simulink model "opalWebSrvExp"  (Simulink 7.8)
settings: Solver=ode4  SolverMode=SingleTasking  StartTime=0  StopTime=inf  FixedStep=Tsrt  MaxStep=0.01  RelTol=1e-3  AbsTol=1e-6
PreLoadFcn:
  | Tsrt=5e-5;
  | Tscom=1e-2;
undefined symbols (not defined in the file): another_event_name, IP, my_event_name, UDP
libraries: rtlab x7, rtio_opalrt_op5142ex1 x5, rtio_generic_ip x1, powerlib_extras x1
settings Model: Creator=jwu  LastModifiedBy=Administrateur  ExtModeTrigMode=oneshot  ExtModeArmWhenConnect=off  BufferReuse=off
settings DataIOCC: ExternalInput=[]  InitialState=[]  LimitDataPoints=off  SaveOutput=off  SaveTime=off  SignalLoggingName=sigsOut
settings OptimizationCC: BooleanDataType=off  OptimizeBlockIOStorage=off  BufferReuse=off  ExpressionFolding=off  FoldNonRolledExpr=off  LocalBlockOutputs=off  InitFltsAndDblsToZero=on
settings DebuggingCC: SaveWithParameterizedLinksMsg=none  SignalResolutionControl=TryResolveAllWithWarning  SolverPrmCheckMsg=none  InheritedTsInSrcMsg=none  MultiTaskDSMMsg=warning  MultiTaskCondExecSysMsg=none  FcnCallInpInsideContextMsg=Use local settings  StrictBusMsg=None
settings HardwareCC: TargetUnknown=on
settings RTWCC: IncludeERTFirstTime=on
settings CodeAppCC: IgnoreCustomStorageClasses=off
settings GRTTargetCC: TargetFcnLib=ansi_tfl_tmw.mat

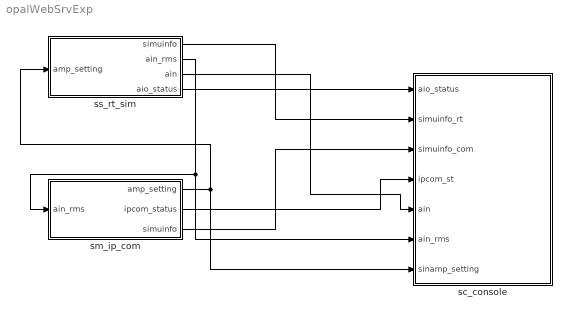
== system opalWebSrvExp ==
  sc_console : Subsystem
  sm_ip_com : Subsystem
  ss_rt_sim : Subsystem
  wires:
  ss_rt_sim/1(simuinfo) -> sc_console/2(simuinfo_rt)
  sm_ip_com/3(simuinfo) -> sc_console/3(simuinfo_com)
  ss_rt_sim/2(ain_rms) -> sm_ip_com/1(ain_rms), sc_console/6(ain_rms)
  sm_ip_com/1(amp_setting) -> ss_rt_sim/1(amp_setting), sc_console/7(sinamp_setting)
  ss_rt_sim/4(aio_status) -> sc_console/1(aio_status)
  sm_ip_com/2(ipcom_status) -> sc_console/4(ipcom_st)
  ss_rt_sim/3(ain) -> sc_console/5(ain)

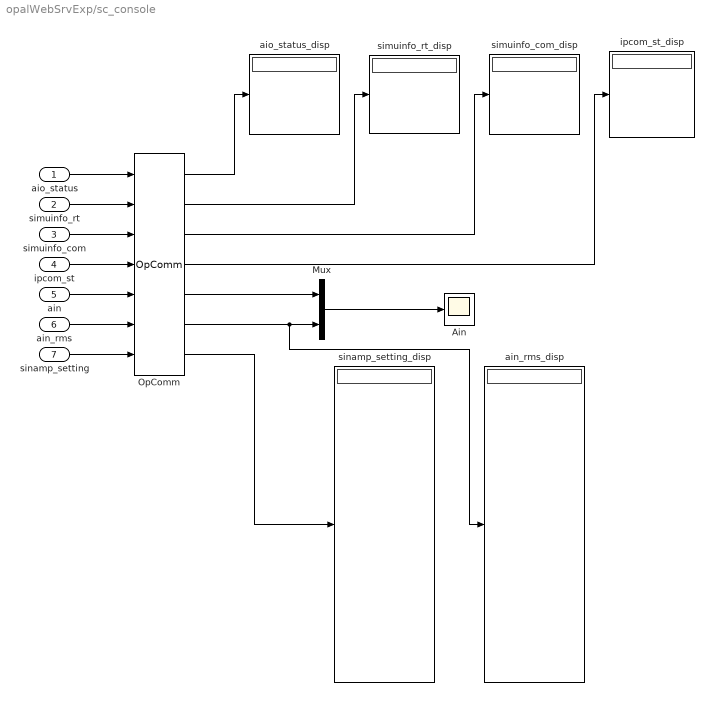
== system opalWebSrvExp/sc_console ==
  aio_status : Inport
  simuinfo_rt : Inport  Port=2
  simuinfo_com : Inport  Port=3
  ipcom_st : Inport  Port=4
  ain : Inport  Port=5
  ain_rms : Inport  Port=6
  sinamp_setting : Inport  Port=7
  Ain : Scope
  Mux : Mux  Inputs=2
  OpComm : rtlab/OpComm  nbport=7  groupe_acq=1  subsys_rate=0  st=0  Synchronization=on  Interpolation=on  Threshold=1.0  Missed_Data=off  Sim_Time=off  Samples=off  dynSigOut=off  from_console=0  warning_done=off  writeOpCommFile=off  Offset=off
  ain_rms_disp : Display
  aio_status_disp : Display
  ipcom_st_disp : Display
  simuinfo_com_disp : Display
  simuinfo_rt_disp : Display
  sinamp_setting_disp : Display
  wires:
  aio_status/1 -> OpComm/1
  ain/1 -> OpComm/5
  OpComm/1 -> aio_status_disp/1
  simuinfo_rt/1 -> OpComm/2
  simuinfo_com/1 -> OpComm/3
  OpComm/2 -> simuinfo_rt_disp/1
  OpComm/3 -> simuinfo_com_disp/1
  ipcom_st/1 -> OpComm/4
  OpComm/4 -> ipcom_st_disp/1
  ain_rms/1 -> OpComm/6
  OpComm/5 -> Mux/1
  OpComm/6 -> Mux/2, ain_rms_disp/1
  Mux/1 -> Ain/1
  sinamp_setting/1 -> OpComm/7
  OpComm/7 -> sinamp_setting_disp/1

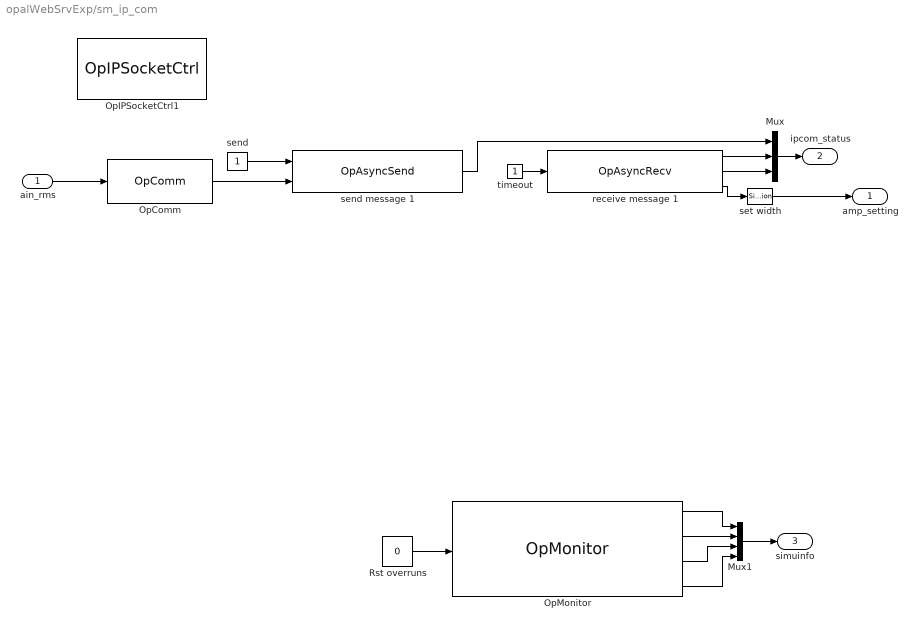
== system opalWebSrvExp/sm_ip_com ==
  ain_rms : Inport
  Mux : Mux  Inputs=3
  Mux1 : Mux
  OpComm : rtlab/OpComm  nbport=1  groupe_acq=1  subsys_rate=Tscom  st=Tscom  Synchronization=on  Interpolation=on  Threshold=1.0  Missed_Data=off  Sim_Time=off  Samples=off  dynSigOut=off  from_console=0  warning_done=off  writeOpCommFile=off  Offset=off
  OpIPSocketCtrl1 : rtio_generic_ip/OpIPSocketCtrl  ctl_id=1  proto=UDP/IP  ip_addr_remote=195.220.18.3  ip_port_remote=50000  ip_port_local=0  ip_addr_mcast=0.0.0.0  exe_name=AsyncIP
  OpMonitor : rtlab/Monitoring/OpMonitor  compute_time=on  real_step=on  idle_time=on  nb_overruns=on  user_time=off  user_name=my_event_name,another_event_name
  Rst overruns : Constant  Value=0
  receive message 1 : rtlab/Communication/Asynchronous/OpAsyncRecv  ctl_id=1  recv_id=1  enable_param=off  fp1=1  fp2=2  fp3=3  fp4=4  fp5=5  sp1=string1  sp2=string2  sp3=string3  sp4=string4  sp5=string5
  send : Constant
  send message 1 : rtlab/Communication/Asynchronous/OpAsyncSend  ctl_id=1  send_id=1  mode=DONT_NEED_REPLY  enable_param=off  fp1=1  fp2=2  fp3=3  fp4=4  fp5=5  sp1=string1  sp2=string2  sp3=string3  sp4=string4  sp5=string5
  set width : SignalSpecification  Dimensions=16
  timeout : Constant
  amp_setting : Outport
  ipcom_status : Outport  Port=2
  simuinfo : Outport  Port=3
  wires:
  receive message 1/3 -> set width/1
  receive message 1/1 -> Mux/2
  receive message 1/2 -> Mux/3
  timeout/1 -> receive message 1/1
  send message 1/1 -> Mux/1
  Mux/1 -> ipcom_status/1
  set width/1 -> amp_setting/1
  ain_rms/1 -> OpComm/1
  OpComm/1 -> send message 1/2
  OpMonitor/1 -> Mux1/1
  OpMonitor/2 -> Mux1/2
  OpMonitor/3 -> Mux1/3
  OpMonitor/4 -> Mux1/4
  Mux1/1 -> simuinfo/1
  Rst overruns/1 -> OpMonitor/1
  send/1 -> send message 1/1

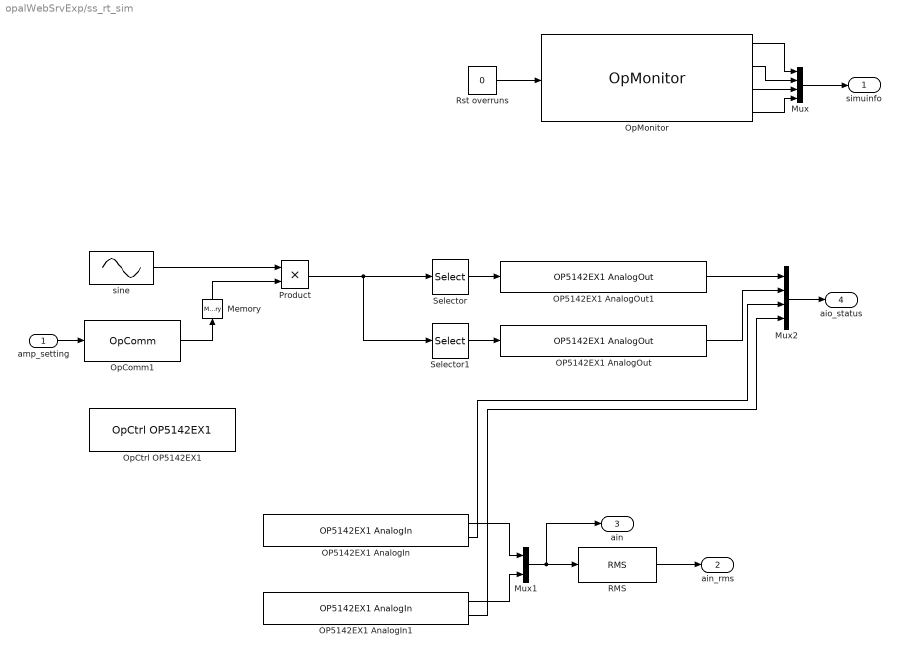
== system opalWebSrvExp/ss_rt_sim ==
  amp_setting : Inport
  Memory : Memory
  Mux : Mux
  Mux1 : Mux  Inputs=2
  Mux2 : Mux
  OP5142EX1 AnalogIn : rtio_opalrt_op5142ex1/OP5142EX1 AnalogIn  CtrlName='OP5142EX1 Ctrl'  portNb=5  FcnNos=Slot 1 Module B Subsection 1  size=16  maxcount=8  count=8  numchan=8  sampleTime=0
      settings: AttributesFormatString=%<CtrlName>
  OP5142EX1 AnalogIn1 : rtio_opalrt_op5142ex1/OP5142EX1 AnalogIn  CtrlName='OP5142EX1 Ctrl'  portNb=6  FcnNos=Slot 1 Module B Subsection 2  size=16  maxcount=8  count=8  numchan=8  sampleTime=0
      settings: AttributesFormatString=%<CtrlName>
  OP5142EX1 AnalogOut : rtio_opalrt_op5142ex1/OP5142EX1 AnalogOut  CtrlName='OP5142EX1 Ctrl'  portNb=2  FcnNos=Slot 1 Module A Subsection 2  size=16  maxcount=8  count=8  numchan=8  israngeinput=off  voltagerange=[-16 ... 16]  slot=0  side=0  mismatch=0  slotside=Slot_1_Module_A
      settings: AttributesFormatString=%<CtrlName>
  OP5142EX1 AnalogOut1 : rtio_opalrt_op5142ex1/OP5142EX1 AnalogOut  CtrlName='OP5142EX1 Ctrl'  portNb=1  FcnNos=Slot 1 Module A Subsection 1  size=16  maxcount=8  count=8  numchan=8  israngeinput=off  voltagerange=[-16 ... 16]  slot=0  side=0  mismatch=0  slotside=Slot_1_Module_A
      settings: AttributesFormatString=%<CtrlName>
  OpComm1 : rtlab/OpComm  nbport=1  groupe_acq=1  subsys_rate=Tsrt  st=Tscom  Synchronization=on  Interpolation=on  Threshold=1.0  Missed_Data=off  Sim_Time=off  Samples=off  dynSigOut=off  from_console=0  warning_done=off  writeOpCommFile=off  Offset=off
  OpCtrl OP5142EX1 : rtio_opalrt_op5142ex1/OpCtrl OP5142EX1  CtrlName='OP5142EX1 Ctrl'  boardid=0  BitstreamFilename=OP5142_1-EX-0000-2_1_3_57-OP5142_8DIO_8TSDIO_6QEIO_16AIO-01-01.bin  numconfig=-1  mode=Master  externalClock=off  decimRtsi=0  calibIO=off  SampleTime=0  loadinport=-1
  OpMonitor : rtlab/Monitoring/OpMonitor  compute_time=on  real_step=on  idle_time=on  nb_overruns=on  user_time=off  user_name=my_event_name,another_event_name
  Product : Product  RndMeth=Zero
  RMS : powerlib_extras/Measurements/RMS  f1=50
  Rst overruns : Constant  Value=0
  Selector : Selector  InputPortWidth=16  IndexOptions=Index vector (dialog)  Indices=[1:8]  OutputSizes=1
  Selector1 : Selector  InputPortWidth=16  IndexOptions=Index vector (dialog)  Indices=[9:16]  OutputSizes=1
  sine : Sin  Frequency=50*2*pi
  simuinfo : Outport
  ain_rms : Outport  Port=2
  ain : Outport  Port=3
  aio_status : Outport  Port=4
  wires:
  sine/1 -> Product/1
  amp_setting/1 -> OpComm1/1
  OpComm1/1 -> Memory/1
  Rst overruns/1 -> OpMonitor/1
  Mux/1 -> simuinfo/1
  OpMonitor/1 -> Mux/1
  OpMonitor/2 -> Mux/2
  OpMonitor/3 -> Mux/3
  OpMonitor/4 -> Mux/4
  Selector/1 -> OP5142EX1 AnalogOut1/1
  Selector1/1 -> OP5142EX1 AnalogOut/1
  Product/1 -> Selector/1, Selector1/1
  OP5142EX1 AnalogIn/1 -> Mux1/1
  OP5142EX1 AnalogIn1/1 -> Mux1/2
  Mux1/1 -> RMS/1, ain/1
  RMS/1 -> ain_rms/1
  OP5142EX1 AnalogOut1/1 -> Mux2/1
  OP5142EX1 AnalogOut/1 -> Mux2/2
  OP5142EX1 AnalogIn/2 -> Mux2/3
  OP5142EX1 AnalogIn1/2 -> Mux2/4
  Mux2/1 -> aio_status/1
  Memory/1 -> Product/2
